simulink library "FaultDetector"  (R2019b)
settings: Solver=VariableStepAuto  StartTime=0.0  StopTime=10.0  RelTol=1e-3
libraries: SampleTime x1
settings Model: Creator=Nick  LastModifiedBy=bashh
settings DataIOCC: ReturnWorkspaceOutputs=off
settings DebuggingCC: ArithmeticOperatorsInVariantConditions=warning
settings SFSimCC: CustomCodeUndefinedFunction=UseInterfaceOnly

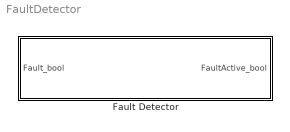
== system FaultDetector ==
  Fault Detector : Subsystem  mask{timeTrip=1, timeReset=1, isSticky=off}
      mask prompts: timeTrip "Time to Trip (s):"; timeReset "Time to Reset (s):"; isSticky "Sticky Fault"
      mask Display:
      | color('blue');
      | 
      | prompt = 'Fault Detector';
      | 
      | if (isSticky)
      |     prompt = [prompt, '\n(Sticky)'];
      |     prompt = [prompt, '\nTrip Time: ', num2str(timeTrip), 's'];
      | else
      |     prompt = [prompt, '\n(Resettable)'];
      |     prompt = [prompt, '\nTrip Time: ', num2str(timeTrip), 's'];
      |     prompt = [prompt, '\nReset Time: ', num2str(timeReset), 's'];
      | end
      | 
      | 
      | 
      | disp(sprintf(prompt));

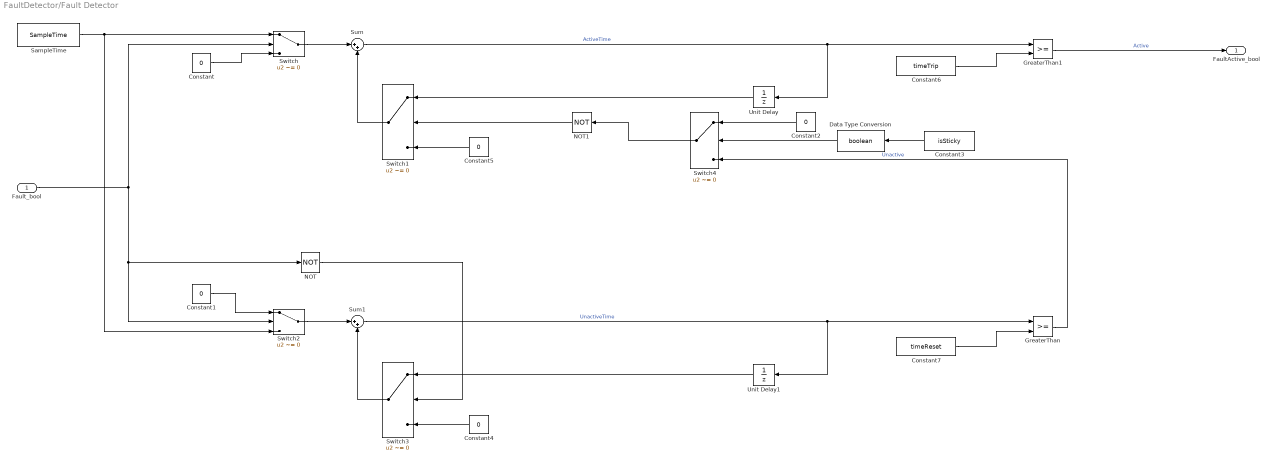
== system FaultDetector/Fault Detector ==
  Fault_bool : Inport  OutDataTypeStr=boolean
  Constant{,1..2,4..5} (5 alike) : Constant  Value=0
  Constant3 : Constant  Value=isSticky
  Constant6 : Constant  Value=timeTrip
  Constant7 : Constant  Value=timeReset
  Data Type Conversion : DataTypeConversion  OutDataTypeStr=boolean
  GreaterThan : RelationalOperator  OutDataTypeStr=boolean  RndMeth=Simplest
  GreaterThan1 : RelationalOperator  OutDataTypeStr=boolean  RndMeth=Simplest
  NOT : Logic  Operator=NOT  IconShape=distinctive  AllPortsSameDT=off  OutDataTypeStr=boolean
  NOT1 : Logic  Operator=NOT  IconShape=distinctive  AllPortsSameDT=off  OutDataTypeStr=boolean
  SampleTime : SampleTime/Algroithms/SampleTime  SystemSampleTime=-1  Latency=0  AutoFrameSizeCalculation=off
  Sum : Sum  Inputs=|++
  Sum1 : Sum  Inputs=|++
  Switch{,1..4} (5 alike) : Switch  Criteria=u2 ~= 0
  Unit Delay : UnitDelay  SampleTime=-1  HasFrameUpgradeWarning=on
  Unit Delay1 : UnitDelay  SampleTime=-1  HasFrameUpgradeWarning=on
  FaultActive_bool : Outport  OutDataTypeStr=boolean
  wires:
  Switch/1 -> Sum/1
  Constant/1 -> Switch/3
  Switch1/1 -> Sum/2
  Sum/1 -> GreaterThan1/1, Unit Delay/1  "ActiveTime"
  Unit Delay/1 -> Switch1/1
  Sum1/1 -> GreaterThan/1, Unit Delay1/1  "UnactiveTime"
  Unit Delay1/1 -> Switch3/1
  Constant1/1 -> Switch2/1
  Switch2/1 -> Sum1/1
  Switch3/1 -> Sum1/2
  SampleTime/1 -> Switch2/3, Switch/1
  NOT/1 -> Switch3/2
  Constant7/1 -> GreaterThan/2
  Constant6/1 -> GreaterThan1/2
  GreaterThan1/1 -> FaultActive_bool/1  "Active"
  GreaterThan/1 -> Switch4/3  "Unactive"
  Constant4/1 -> Switch3/3
  Constant5/1 -> Switch1/3
  NOT1/1 -> Switch1/2
  Fault_bool/1 -> NOT/1, Switch2/2, Switch/2
  Switch4/1 -> NOT1/1
  Constant2/1 -> Switch4/1
  Constant3/1 -> Data Type Conversion/1
  Data Type Conversion/1 -> Switch4/2
